simulink model "untitled"  (R2020a)
settings: Solver=VariableStepAuto  StartTime=0.0  StopTime=30  RelTol=1e-3
settings Model: Creator=nose  LastModifiedBy=nose

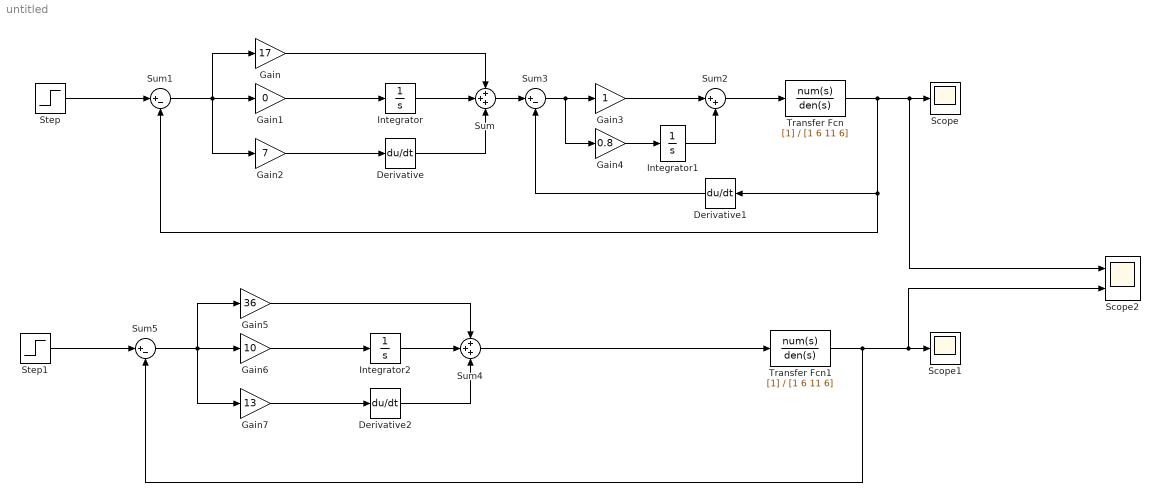
== system untitled ==
  Derivative : Derivative
  Derivative1 : Derivative
  Derivative2 : Derivative
  Gain : Gain  Gain=17
  Gain1 : Gain  Gain=0
  Gain2 : Gain  Gain=7
  Gain3 : Gain
  Gain4 : Gain  Gain=0.8
  Gain5 : Gain  Gain=36
  Gain6 : Gain  Gain=10
  Gain7 : Gain  Gain=13
  Integrator : Integrator
  Integrator1 : Integrator
  Integrator2 : Integrator
  Scope : Scope
  Scope1 : Scope
  Scope2 : Scope  NumInputPorts=2
  Step : Step  Time=3  After=100  SampleTime=0
  Step1 : Step  Time=3  After=100  SampleTime=0
  Sum : Sum  Inputs=+++
  Sum1 : Sum  Inputs=|+-
  Sum2 : Sum  Inputs=|++
  Sum3 : Sum  Inputs=|+-
  Sum4 : Sum  Inputs=+++
  Sum5 : Sum  Inputs=|+-
  Transfer Fcn : TransferFcn  Denominator=[1 6 11 6]
  Transfer Fcn1 : TransferFcn  Denominator=[1 6 11 6]
  wires:
  Gain2/1 -> Derivative/1
  Gain1/1 -> Integrator/1
  Integrator/1 -> Sum/2
  Derivative/1 -> Sum/3
  Gain/1 -> Sum/1
  Transfer Fcn/1 -> Scope2/1, Scope/1, Derivative1/1, Sum1/2
  Sum1/1 -> Gain2/1, Gain/1, Gain1/1
  Step/1 -> Sum1/1
  Gain4/1 -> Integrator1/1
  Gain3/1 -> Sum2/1
  Integrator1/1 -> Sum2/2
  Sum2/1 -> Transfer Fcn/1
  Sum3/1 -> Gain4/1, Gain3/1
  Derivative1/1 -> Sum3/2
  Sum/1 -> Sum3/1
  Step1/1 -> Sum5/1
  Transfer Fcn1/1 -> Scope1/1, Scope2/2, Sum5/2
  Sum5/1 -> Gain7/1, Gain5/1, Gain6/1
  Integrator2/1 -> Sum4/2
  Gain7/1 -> Derivative2/1
  Gain6/1 -> Integrator2/1
  Derivative2/1 -> Sum4/3
  Gain5/1 -> Sum4/1
  Sum4/1 -> Transfer Fcn1/1
